simulink model "sim1"  (R2013a)
settings: Solver=ode4  StartTime=0.0  StopTime=10.0  FixedStep=0.1  RelTol=1e-3
undefined symbols (not defined in the file): c
settings Model: Creator=nyquist  LastModifiedBy=nyquist

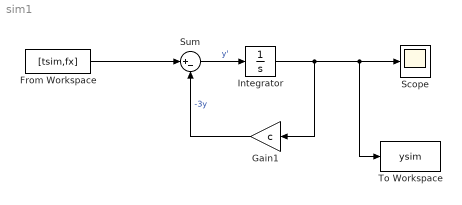
== system sim1 ==
  From Workspace : FromWorkspace  VariableName=[tsim,fx]  SampleTime=0.1  Interpolate=off  OutputAfterFinalValue=Setting to zero
  Gain1 : Gain  Gain=c
  Integrator : Integrator
  Scope : Scope
  Sum : Sum  Inputs=|+-
  To Workspace : ToWorkspace  VariableName=ysim  SampleTime=0.1
  wires:
  From Workspace/1 -> Sum/1
  Gain1/1 -> Sum/2  "-3y"
  Sum/1 -> Integrator/1  "y'"
  Integrator/1 -> Gain1/1, To Workspace/1, Scope/1
